simulink model "SLSingleLink_Begin"  (R2014b)
settings: Solver=ode45  StartTime=0.0  StopTime=2*pi  RelTol=1e-3
PreLoadFcn:
  | g = 9.81;
  | rho = 1;
  | m = 1;
  | b = 1;
settings Model: Creator=cosorio  LastModifiedBy=cosorio
settings DataIOCC: LimitDataPoints=off  SignalLoggingSaveFormat=ModelDataLogs  SaveTime=off
settings OptimizationCC: ExpressionDepthLimit=2147483647
settings DebuggingCC: UnderspecifiedInitializationDetection=Classic  MergeDetectMultiDrivingBlocksExec=none  SolverPrmCheckMsg=none  FcnCallInpInsideContextMsg=UseLocalSettings  StateNameClashWarn=warning
settings GRTTargetCC: CombineOutputUpdateFcns=off  GRTInterface=on

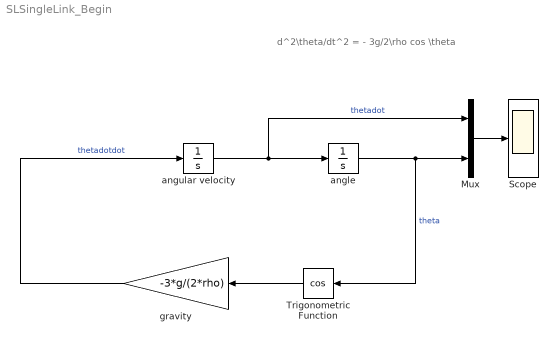
== system SLSingleLink_Begin ==
  note: d^2\theta/dt^2 = - 3g/2\rho cos \theta
  Mux : Mux  Inputs=2
  Scope : Scope
      settings: ShowLegends=on  YMin=-10  YMax=10
  Trigonometric Function : Trigonometry  Operator=cos
  angle : Integrator  InitialCondition=45*pi/180
  angular velocity : Integrator
  gravity : Gain  Gain=-3*g/(2*rho)
  wires:
  angle/1 -> Mux/2, Trigonometric Function/1  "theta"
  angular velocity/1 -> Mux/1, angle/1  "thetadot"
  Trigonometric Function/1 -> gravity/1
  gravity/1 -> angular velocity/1  "thetadotdot"
  Mux/1 -> Scope/1
